simulink model "GainAdjustment"  (R2013b)
settings: Solver=ode45  StartTime=0.0  StopTime=100  RelTol=1e-3
settings Model: Creator=MMSA  LastModifiedBy=MMSA
settings SolverCC: ZeroCrossAlgorithm=Adaptive  PositivePriorityOrder=on
settings HardwareCC: ProdBitPerPointer=64  ProdHWDeviceType=Generic->64-bit Embedded Processor (LLP64)

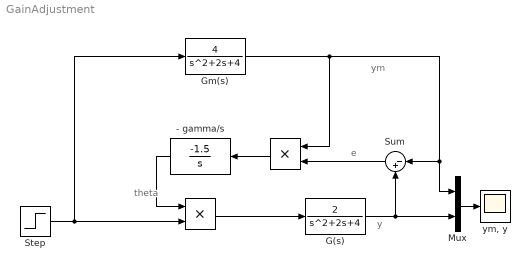
== system GainAdjustment ==
  note: theta
  note: e
  note: ym
  note: y
  " " : Product
  "  " : Product
  "- gamma/s " : TransferFcn  Numerator=[-1.5]  Denominator=[1 0]
  G(s) : TransferFcn  Numerator=[2]  Denominator=[1 2 4]
  Gm(s) : TransferFcn  Numerator=[4]  Denominator=[1 2 4]
  Mux : Mux  Inputs=2
  Step : Step  Time=0  SampleTime=0
  Sum : Sum  Inputs=|-+
  "ym, y" : Scope
  wires:
  G(s)/1 -> Sum/2, Mux/2
  Gm(s)/1 -> Sum/1, Mux/1, " "/1
  Sum/1 -> " "/2
  " "/1 -> "- gamma/s "/1
  "  "/1 -> G(s)/1
  Step/1 -> Gm(s)/1, "  "/2
  "- gamma/s "/1 -> "  "/1
  Mux/1 -> "ym, y"/1
